simulink model "test_r2_snapshot"  (Simulink 7.9)
settings: Solver=ode45  StartTime=0.0  StopTime=10.0  RelTol=1e-3
libraries: xbsIndex_r4 x545, xps_library x13, casper_library_misc x4, casper_library_scopes x2
(part 1 of 4)
settings Model: Creator=jmanley  LastModifiedBy=jmanley

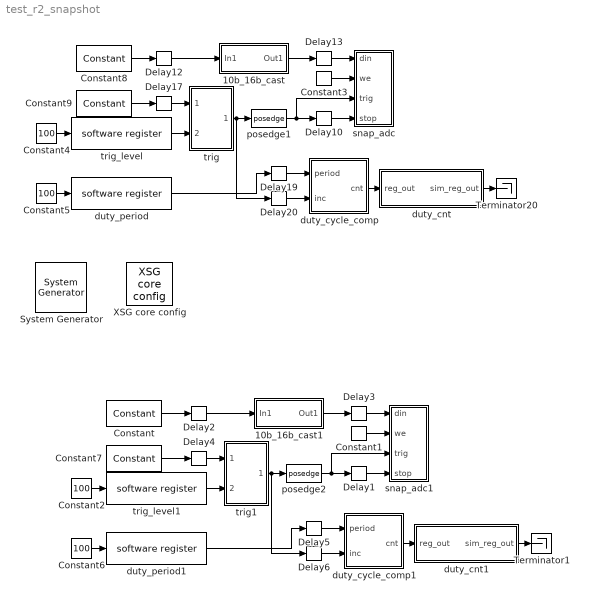
== system test_r2_snapshot ==
  " System Generator" : xbsIndex_r4/ System Generator  Tag=genX  xilinxfamily=virtex5  part=xc5vsx95t  speed=-1  package=ff1136  synthesis_tool=XST  clock_wrapper=Clock Enables  directory=./test_ratt2_snapshot/sysgen  proj_type=Project Navigator  Synth_file=XST Defaults  Impl_file=ISE Defaults  testbench=off  simulink_period=1  sysclk_period=5  dcm_input_clock_period=100  incr_netlist=off  trim_vbits=Everywhere in SubSystem  dbl_ovrd=According to Block Masks  core_generation=According to Block Masks  run_coregen=off  deprecated_control=off  eval_field=0  block_type=sysgen
      settings: block_version=11.4
  10b_16b_cast : Subsystem
  10b_16b_cast1 : Subsystem
  Constant : xbsIndex_r4/Constant  const=0  gui_display_data_type=Fixed-point  arith_type=Unsigned  n_bits=80  bin_pt=0  preci_type=Single  exp_width=8  frac_width=24  explicit_period=on  period=1  equ=P=C  opselect=C  inp2=PCIN>>17  opr=+  inp1=P  carry=CIN  dbl_ovrd=off  block_type=constant
      settings: block_version=11.4
  Constant1 : xbsIndex_r4/Constant  const=1  gui_display_data_type=Fixed-point  arith_type=Boolean  n_bits=1  bin_pt=0  preci_type=Single  exp_width=8  frac_width=24  explicit_period=off  period=1  equ=P=C  opselect=C  inp2=PCIN>>17  opr=+  inp1=P  carry=CIN  dbl_ovrd=off  block_type=constant
      settings: block_version=11.4
  Constant{2,4..6} (4 alike) : Constant  Value=100
  Constant3 : xbsIndex_r4/Constant  const=1  gui_display_data_type=Fixed-point  arith_type=Boolean  n_bits=1  bin_pt=0  preci_type=Single  exp_width=8  frac_width=24  explicit_period=off  period=1  equ=P=C  opselect=C  inp2=PCIN>>17  opr=+  inp1=P  carry=CIN  dbl_ovrd=off  block_type=constant
      settings: block_version=11.4
  Constant7 : xbsIndex_r4/Constant  const=0  gui_display_data_type=Fixed-point  arith_type=Unsigned  n_bits=80  bin_pt=0  preci_type=Single  exp_width=8  frac_width=24  explicit_period=on  period=1  equ=P=C  opselect=C  inp2=PCIN>>17  opr=+  inp1=P  carry=CIN  dbl_ovrd=off  block_type=constant
      settings: block_version=11.4
  Constant8 : xbsIndex_r4/Constant  const=(2^80)-1  gui_display_data_type=Fixed-point  arith_type=Unsigned  n_bits=80  bin_pt=0  preci_type=Single  exp_width=8  frac_width=24  explicit_period=on  period=1  equ=P=C  opselect=C  inp2=PCIN>>17  opr=+  inp1=P  carry=CIN  dbl_ovrd=off  block_type=constant
      settings: block_version=11.4
  Constant9 : xbsIndex_r4/Constant  const=(2^80)-1  gui_display_data_type=Fixed-point  arith_type=Unsigned  n_bits=80  bin_pt=0  preci_type=Single  exp_width=8  frac_width=24  explicit_period=on  period=1  equ=P=C  opselect=C  inp2=PCIN>>17  opr=+  inp1=P  carry=CIN  dbl_ovrd=off  block_type=constant
      settings: block_version=11.4
  Delay{1..6,10,12..13,17,19..20} (12 alike) : xbsIndex_r4/Delay  rst=off  infoeditControl=Selection of Reset will increase slice count due to use of real FFs and instead of SRLs  en=off  latency=2  dbl_ovrd=off  reg_retiming=on  block_type=delay
  Terminator1 : Terminator
  Terminator20 : Terminator
  XSG core config : xps_library/XSG core config  Tag=xps:xsg  hw_sys=ROACH2:sx475t  clk_src=sys_clk  ROACH_clk_src=sys_clk2x  ROACH2_clk_src=sys_clk  clk_rate=225  sample_period=1  synthesis_tool=XST
  duty_cnt : Subsystem  Tag=xps:sw_reg  mask{io_dir=To Processor, arith_type=Unsigned, bitwidth=32, bin_pt=0, sample_period=1, latency=0}
      mask prompts: io_dir "I/O direction"; arith_type "Data Type"; bitwidth "Data bitwidth"; bin_pt "Data binary point"; sample_period "Sample period"
      mask init:
      | gw_name = clear_name(gcb);
      | config.source = str2func('software_register_init');
      | config.toplevel = gcb;
      | xBlock( config, {io_dir, arith_type, bitwidth, bin_pt, ... 
      |     sample_period, gw_name, latency});
      mask StyleString: popup(From Processor|To Processor),popup(Unsigned|Signed  (2's comp)),edit,edit,edit,edit
  duty_cnt1 : Subsystem  Tag=xps:sw_reg  mask{io_dir=To Processor, arith_type=Unsigned, bitwidth=32, bin_pt=0, sample_period=1, latency=0}
      mask prompts: io_dir "I/O direction"; arith_type "Data Type"; bitwidth "Data bitwidth"; bin_pt "Data binary point"; sample_period "Sample period"
      mask init:
      | gw_name = clear_name(gcb);
      | config.source = str2func('software_register_init');
      | config.toplevel = gcb;
      | xBlock( config, {io_dir, arith_type, bitwidth, bin_pt, ... 
      |     sample_period, gw_name, latency});
      mask StyleString: popup(From Processor|To Processor),popup(Unsigned|Signed  (2's comp)),edit,edit,edit,edit
  duty_cycle_comp : Subsystem  mask{chan_bits=12}
      mask prompts: chan_bits "Number of Channels (2^?)"
  duty_cycle_comp1 : Subsystem  mask{chan_bits=12}
      mask prompts: chan_bits "Number of Channels (2^?)"
  duty_period : xps_library/software register  Tag=xps:sw_reg  io_dir=From Processor  arith_type=Unsigned  bitwidth=32  bin_pt=0  sample_period=1  gw_name=test_ratt2_snapshot_duty_period_user_data_out
  duty_period1 : xps_library/software register  Tag=xps:sw_reg  io_dir=From Processor  arith_type=Unsigned  bitwidth=32  bin_pt=0  sample_period=1  gw_name=test_ratt2_snapshot_duty_period1_user_data_out
  posedge1 : casper_library_misc/posedge  Tag=Rising Edge Detector
  posedge2 : casper_library_misc/posedge  Tag=Rising Edge Detector
  snap_adc : Subsystem  AncestorBlock=casper_library_scopes/snapshot  mask(snapshot){storage=bram, dram_dimm=1, dram_clock=200, nsamples=12, data_width=128, offset=on, circap=on, value=off, use_dsp48=on}
      mask prompts: storage "Storage medium"; dram_dimm "DRAM dimm"; dram_clock "DRAM clock rate"; nsamples "Number of Samples (2^?)"; data_width "Data width"; offset "Start delay support"; circap "Circular capture support"; value "Extra value capture support"; use_dsp48 "Use DSP48s to implement counters"
      mask help:
      | Standard snap block, but with the following optional extras;
      |  1) Optionally delay the fabric trigger by a user-specified number of valids.
      |  2) Capture continuously after a trigger until a stop pulse is received. Data is captured into BRAM continuously, with old data being overwritten until a stop command is received. Then stop capturing when memory is filled. This enables you to get some data before and some data after the stop pulse. Use the 'tr_en_cnt' register to determine where you are in your vector. 'Addr' register's MSb now indicates 'busy capturing'.
      |  3) Optionally capture a value on an input port to a register at the same time as the first data sample.
      |  4) Implement counters using DSP48Es to save resources.
      mask init:
      | snapshot_init(gcb, ...
      |     'storage', storage, ...
      |     'dram_dimm', dram_dimm, ...
      |     'dram_clock', dram_clock, ...
      |     'nsamples', nsamples, ...
      |     'data_width', data_width, ...
      |     'offset', offset, ...
      |     'circap', circap, ...
      |     'value', value, ...
      |     'use_dsp48', use_dsp48);
      mask StyleString: popup(bram|dram),popup(1|2|3|4),popup(200|250|266|300|333),edit,popup(8|16|32|64|128),checkbox,checkbox,checkbox,checkbox
      mask CallbackString: snapshot_callback();||||||||
  snap_adc1 : Subsystem  AncestorBlock=casper_library_scopes/snapshot  mask(snapshot){storage=bram, dram_dimm=1, dram_clock=200, nsamples=12, data_width=128, offset=on, circap=on, value=off, use_dsp48=on}
      mask prompts: storage "Storage medium"; dram_dimm "DRAM dimm"; dram_clock "DRAM clock rate"; nsamples "Number of Samples (2^?)"; data_width "Data width"; offset "Start delay support"; circap "Circular capture support"; value "Extra value capture support"; use_dsp48 "Use DSP48s to implement counters"
      mask help:
      | Standard snap block, but with the following optional extras;
      |  1) Optionally delay the fabric trigger by a user-specified number of valids.
      |  2) Capture continuously after a trigger until a stop pulse is received. Data is captured into BRAM continuously, with old data being overwritten until a stop command is received. Then stop capturing when memory is filled. This enables you to get some data before and some data after the stop pulse. Use the 'tr_en_cnt' register to determine where you are in your vector. 'Addr' register's MSb now indicates 'busy capturing'.
      |  3) Optionally capture a value on an input port to a register at the same time as the first data sample.
      |  4) Implement counters using DSP48Es to save resources.
      mask init: same as test_r2_snapshot/snap_adc
      mask StyleString: popup(bram|dram),popup(1|2|3|4),popup(200|250|266|300|333),edit,popup(8|16|32|64|128),checkbox,checkbox,checkbox,checkbox
      mask CallbackString: snapshot_callback();||||||||
  trig : Subsystem
  trig1 : Subsystem
  trig_level : xps_library/software register  Tag=xps:sw_reg  io_dir=From Processor  arith_type=Unsigned  bitwidth=32  bin_pt=0  sample_period=1  gw_name=test_ratt2_snapshot_trig_level_user_data_out
  trig_level1 : xps_library/software register  Tag=xps:sw_reg  io_dir=From Processor  arith_type=Unsigned  bitwidth=32  bin_pt=0  sample_period=1  gw_name=test_ratt2_snapshot_trig_level1_user_data_out
  wires:
  Constant4/1 -> trig_level/1
  Constant9/1 -> Delay17/1
  trig/1(trig) -> posedge1/1, Delay20/1
  trig_level/1 -> trig/2(trig_pnt)
  Delay17/1 -> trig/1(adc_data)
  posedge1/1 -> Delay10/1, snap_adc/3(trig)
  Delay10/1 -> snap_adc/4(stop)
  Constant5/1 -> duty_period/1
  duty_period/1 -> Delay19/1
  duty_cnt/1(sim_reg_out) -> Terminator20/1
  duty_cycle_comp/1(cnt) -> duty_cnt/1(reg_out)
  Delay19/1 -> duty_cycle_comp/1(period)
  Delay20/1 -> duty_cycle_comp/2(inc)
  Constant3/1 -> snap_adc/2(we)
  Constant8/1 -> Delay12/1
  Delay12/1 -> 10b_16b_cast/1(In1)
  10b_16b_cast/1(Out1) -> Delay13/1
  Delay13/1 -> snap_adc/1(din)
  Constant2/1 -> trig_level1/1
  Constant7/1 -> Delay4/1
  trig1/1(trig) -> Delay6/1, posedge2/1
  trig_level1/1 -> trig1/2(trig_pnt)
  Delay4/1 -> trig1/1(adc_data)
  posedge2/1 -> snap_adc1/3(trig), Delay1/1
  Delay1/1 -> snap_adc1/4(stop)
  Constant6/1 -> duty_period1/1
  duty_period1/1 -> Delay5/1
  duty_cnt1/1(sim_reg_out) -> Terminator1/1
  duty_cycle_comp1/1(cnt) -> duty_cnt1/1(reg_out)
  Delay5/1 -> duty_cycle_comp1/1(period)
  Delay6/1 -> duty_cycle_comp1/2(inc)
  Constant1/1 -> snap_adc1/2(we)
  Constant/1 -> Delay2/1
  Delay2/1 -> 10b_16b_cast1/1(In1)
  10b_16b_cast1/1(Out1) -> Delay3/1
  Delay3/1 -> snap_adc1/1(din)

== system test_r2_snapshot/10b_16b_cast ==
  In1 : Inport
  Convert{,1..7} (8 alike) : xbsIndex_r4/Convert  gui_display_data_type=Fixed-point  arith_type="Signed  (2's comp)"  n_bits=16  bin_pt=0  float_type=Single  exp_bits=8  fraction_bits=24  quantization=Truncate  overflow=Wrap  en=off  latency=0  dbl_ovrd=off  pipeline=off  block_type=convert
  adc0_bus_create1 : Subsystem  AncestorBlock=casper_library_flow_control/bus_create  mask(bus_create){inputNum=8}
      mask prompts: inputNum "Number of inputs:"
      mask init:
      | bus_create_init(gcb,...
      |     'inputNum', inputNum);
  bus_expand2 : Subsystem  AncestorBlock=casper_library_flow_control/bus_expand  mask(bus_expand){mode=divisions of equal size, outputNum=8, outputWidth=10, outputBinaryPt=0, outputArithmeticType=1, outputToWorkspace=off, variablePrefix=out, outputToModelAsWell=on}
      mask prompts: outputNum "Number of outputs:"; outputWidth "Output width:"; outputBinaryPt "Output binary point position:"; outputArithmeticType "Output arithmetic type: (Unsigned=0, Signed=1, Boolean=2)"; outputToWorkspace "Output to workspace?"; variablePrefix "Variable name prefix:"; outputToModelAsWell "Output to model as well?"
      mask help:
      | Expands a 'bus' made using a bus_create or Xilinx
      | concat block.
      | The input will be divided into the specified number
      | of outputs with the specified arithmetic types.
      | Divisions are made from most significant bit.
      mask init:
      | bus_expand_init(gcb,...
      |     'mode', mode, ...
      |     'outputNum', outputNum, ...
      |     'outputWidth', outputWidth, ...
      |     'outputBinaryPt', outputBinaryPt, ...
      |     'outputArithmeticType', outputArithmeticType, ...
      |     'outputToWorkspace', outputToWorkspace, ...
      |     'variablePrefix', variablePrefix, ...
      |     'outputToModelAsWell', outputToModelAsWell);
      settings: AttributesFormatString=8 outputs
      mask StyleString: popup(divisions of equal size|divisions of arbitrary size),edit,edit,edit,edit,checkbox,edit,checkbox
      mask CallbackString: bus_expand_callback();||bus_expand_callback();|||bus_expand_callback();||
  Out1 : Outport
  wires:
  bus_expand2/1(msb_out8) -> Convert/1
  bus_expand2/2(out7) -> Convert1/1
  bus_expand2/3(out6) -> Convert2/1
  bus_expand2/4(out5) -> Convert3/1
  bus_expand2/5(out4) -> Convert4/1
  bus_expand2/6(out3) -> Convert5/1
  bus_expand2/7(out2) -> Convert6/1
  bus_expand2/8(lsb_out1) -> Convert7/1
  Convert/1 -> adc0_bus_create1/1(in1)
  Convert1/1 -> adc0_bus_create1/2(in2)
  Convert2/1 -> adc0_bus_create1/3(in3)
  Convert3/1 -> adc0_bus_create1/4(in4)
  Convert4/1 -> adc0_bus_create1/5(in5)
  Convert5/1 -> adc0_bus_create1/6(in6)
  Convert6/1 -> adc0_bus_create1/7(in7)
  Convert7/1 -> adc0_bus_create1/8(in8)
  adc0_bus_create1/1(bus_out) -> Out1/1
  In1/1 -> bus_expand2/1(bus_in)

== system test_r2_snapshot/10b_16b_cast1 ==
  In1 : Inport
  Convert{,1..7} (8 alike) : xbsIndex_r4/Convert  gui_display_data_type=Fixed-point  arith_type="Signed  (2's comp)"  n_bits=16  bin_pt=0  float_type=Single  exp_bits=8  fraction_bits=24  quantization=Truncate  overflow=Wrap  en=off  latency=0  dbl_ovrd=off  pipeline=off  block_type=convert
  adc0_bus_create1 : Subsystem  AncestorBlock=casper_library_flow_control/bus_create  mask(bus_create){inputNum=8}
      mask prompts: inputNum "Number of inputs:"
      mask init:
      | bus_create_init(gcb,...
      |     'inputNum', inputNum);
  bus_expand2 : Subsystem  AncestorBlock=casper_library_flow_control/bus_expand  mask(bus_expand){mode=divisions of equal size, outputNum=8, outputWidth=10, outputBinaryPt=0, outputArithmeticType=1, outputToWorkspace=off, variablePrefix=out, outputToModelAsWell=on}
      mask prompts: outputNum "Number of outputs:"; outputWidth "Output width:"; outputBinaryPt "Output binary point position:"; outputArithmeticType "Output arithmetic type: (Unsigned=0, Signed=1, Boolean=2)"; outputToWorkspace "Output to workspace?"; variablePrefix "Variable name prefix:"; outputToModelAsWell "Output to model as well?"
      mask help:
      | Expands a 'bus' made using a bus_create or Xilinx
      | concat block.
      | The input will be divided into the specified number
      | of outputs with the specified arithmetic types.
      | Divisions are made from most significant bit.
      mask init: same as test_r2_snapshot/10b_16b_cast/bus_expand2
      settings: AttributesFormatString=8 outputs
      mask StyleString: popup(divisions of equal size|divisions of arbitrary size),edit,edit,edit,edit,checkbox,edit,checkbox
      mask CallbackString: bus_expand_callback();||bus_expand_callback();|||bus_expand_callback();||
  Out1 : Outport
  wires:
  In1/1 -> bus_expand2/1(bus_in)
  adc0_bus_create1/1(bus_out) -> Out1/1
  Convert7/1 -> adc0_bus_create1/8(in8)
  Convert6/1 -> adc0_bus_create1/7(in7)
  Convert5/1 -> adc0_bus_create1/6(in6)
  Convert4/1 -> adc0_bus_create1/5(in5)
  Convert3/1 -> adc0_bus_create1/4(in4)
  Convert2/1 -> adc0_bus_create1/3(in3)
  Convert1/1 -> adc0_bus_create1/2(in2)
  Convert/1 -> adc0_bus_create1/1(in1)
  bus_expand2/8(lsb_out1) -> Convert7/1
  bus_expand2/7(out2) -> Convert6/1
  bus_expand2/6(out3) -> Convert5/1
  bus_expand2/5(out4) -> Convert4/1
  bus_expand2/4(out5) -> Convert3/1
  bus_expand2/3(out6) -> Convert2/1
  bus_expand2/2(out7) -> Convert1/1
  bus_expand2/1(msb_out8) -> Convert/1

== system test_r2_snapshot/duty_cnt ==
  reg_out : Inport
  convert : xbsIndex_r4/Convert  gui_display_data_type=Fixed-point  arith_type=Unsigned  n_bits=32  bin_pt=0  float_type=Single  exp_bits=8  fraction_bits=24  quantization=Truncate  overflow=Wrap  en=off  latency=0  dbl_ovrd=off  pipeline=off  block_type=convert
  test_ratt2_snapshot_duty_cnt_user_data_in : xbsIndex_r4/Gateway Out  inherit_from_input=off  hdl_port=on  timing_constraint=None  locs_specified=off  LOCs={}  UseAsDAC=off  DACChannel='1'  block_type=gatewayout
  sim_reg_out : Outport
  wires:
  reg_out/1 -> convert/1
  convert/1 -> test_ratt2_snapshot_duty_cnt_user_data_in/1
  test_ratt2_snapshot_duty_cnt_user_data_in/1 -> sim_reg_out/1

== system test_r2_snapshot/duty_cnt1 ==
  reg_out : Inport
  convert : xbsIndex_r4/Convert  gui_display_data_type=Fixed-point  arith_type=Unsigned  n_bits=32  bin_pt=0  float_type=Single  exp_bits=8  fraction_bits=24  quantization=Truncate  overflow=Wrap  en=off  latency=0  dbl_ovrd=off  pipeline=off  block_type=convert
  test_ratt2_snapshot_duty_cnt1_user_data_in : xbsIndex_r4/Gateway Out  inherit_from_input=off  hdl_port=on  timing_constraint=None  locs_specified=off  LOCs={}  UseAsDAC=off  DACChannel='1'  block_type=gatewayout
  sim_reg_out : Outport
  wires:
  reg_out/1 -> convert/1
  convert/1 -> test_ratt2_snapshot_duty_cnt1_user_data_in/1
  test_ratt2_snapshot_duty_cnt1_user_data_in/1 -> sim_reg_out/1

== system test_r2_snapshot/duty_cycle_comp ==
  period : Inport
  inc : Inport  Port=2
  AddSub : xbsIndex_r4/AddSub  mode=Subtraction  use_carryin=off  use_carryout=off  en=off  latency=1  precision=User Defined  arith_type=Unsigned  n_bits=32  bin_pt=0  quantization=Truncate  overflow=Wrap  dbl_ovrd=off  use_behavioral_HDL=off  hw_selection=DSP48  pipelined=on  block_type=addsub
  Constant2 : xbsIndex_r4/Constant  const=2  gui_display_data_type=Fixed-point  arith_type=Unsigned  n_bits=2  bin_pt=0  preci_type=Single  exp_width=8  frac_width=24  explicit_period=on  period=1  equ=P=C  opselect=C  inp2=PCIN>>17  opr=+  inp1=P  carry=CIN  dbl_ovrd=off  block_type=constant
  Delay1 : xbsIndex_r4/Delay  rst=off  infoeditControl=Selection of Reset will increase slice count due to use of real FFs and instead of SRLs  en=off  latency=1  dbl_ovrd=off  reg_retiming=on  block_type=delay
      settings: xl_area=[0, 0, 0, 0, 0, 0, 0]
  Delay2 : xbsIndex_r4/Delay  rst=off  infoeditControl=Selection of Reset will increase slice count due to use of real FFs and instead of SRLs  en=off  latency=1  dbl_ovrd=off  reg_retiming=on  block_type=delay
      settings: xl_area=[0, 0, 0, 0, 0, 0, 0]
  Register : xbsIndex_r4/Register  init=0  rst=off  en=on  dbl_ovrd=off  block_type=register
      settings: xl_area=[0, 0, 0, 0, 0, 0, 0]
  Relational5 : xbsIndex_r4/Relational  mode=a>=b  en=off  latency=1  dbl_ovrd=off  block_type=relational
      settings: xl_area=[0, 0, 0, 0, 0, 0, 0]  block_version=10.1.3
  Shift : xbsIndex_r4/Shift  shift_dir=Left  shift_bits=chan_bits  en=off  latency=0  precision=Full  arith_type="Signed  (2's comp)"  n_bits=8  bin_pt=2  quantization=Truncate  overflow=Wrap  dbl_ovrd=off  block_type=shift
      settings: xl_area=[0, 0, 0, 0, 0, 0, 0]  block_version=10.1.3
  cntr : xbsIndex_r4/Counter  cnt_type=Free Running  cnt_to=Inf  operation=Up  start_count=1  cnt_by_val=1  arith_type=Unsigned  n_bits=32  bin_pt=0  load_pin=off  rst=on  en=off  explicit_period=on  period=1  dbl_ovrd=off  use_behavioral_HDL=on  implementation=Fabric  use_rpm=on  block_type=counter
      settings: xl_area=[0, 0, 0, 0, 0, 0, 0]
  cntr1 : xbsIndex_r4/Counter  cnt_type=Free Running  cnt_to=Inf  operation=Up  start_count=1  cnt_by_val=1  arith_type=Unsigned  n_bits=32  bin_pt=0  load_pin=off  rst=on  en=on  explicit_period=on  period=1  dbl_ovrd=off  use_behavioral_HDL=on  implementation=Fabric  use_rpm=on  block_type=counter
      settings: xl_area=[0, 0, 0, 0, 0, 0, 0]
  posedge2 : Subsystem  Tag=Rising Edge Detector
  cnt : Outport
  wires:
  Constant2/1 -> AddSub/2
  AddSub/1 -> Delay2/1
  Shift/1 -> AddSub/1
  Delay1/1 -> posedge2/1(In)
  Relational5/1 -> Delay1/1, cntr/1
  period/1 -> Shift/1
  posedge2/1(Out) -> cntr1/1, Register/2
  Delay2/1 -> Relational5/2
  cntr/1 -> Relational5/1
  inc/1 -> cntr1/2
  cntr1/1 -> Register/1
  Register/1 -> cnt/1

== system test_r2_snapshot/duty_cycle_comp1 ==
  period : Inport
  inc : Inport  Port=2
  AddSub : xbsIndex_r4/AddSub  mode=Subtraction  use_carryin=off  use_carryout=off  en=off  latency=1  precision=User Defined  arith_type=Unsigned  n_bits=32  bin_pt=0  quantization=Truncate  overflow=Wrap  dbl_ovrd=off  use_behavioral_HDL=off  hw_selection=DSP48  pipelined=on  block_type=addsub
  Constant2 : xbsIndex_r4/Constant  const=2  gui_display_data_type=Fixed-point  arith_type=Unsigned  n_bits=2  bin_pt=0  preci_type=Single  exp_width=8  frac_width=24  explicit_period=on  period=1  equ=P=C  opselect=C  inp2=PCIN>>17  opr=+  inp1=P  carry=CIN  dbl_ovrd=off  block_type=constant
  Delay1 : xbsIndex_r4/Delay  rst=off  infoeditControl=Selection of Reset will increase slice count due to use of real FFs and instead of SRLs  en=off  latency=1  dbl_ovrd=off  reg_retiming=on  block_type=delay
      settings: xl_area=[0, 0, 0, 0, 0, 0, 0]
  Delay2 : xbsIndex_r4/Delay  rst=off  infoeditControl=Selection of Reset will increase slice count due to use of real FFs and instead of SRLs  en=off  latency=1  dbl_ovrd=off  reg_retiming=on  block_type=delay
      settings: xl_area=[0, 0, 0, 0, 0, 0, 0]
  Register : xbsIndex_r4/Register  init=0  rst=off  en=on  dbl_ovrd=off  block_type=register
      settings: xl_area=[0, 0, 0, 0, 0, 0, 0]
  Relational5 : xbsIndex_r4/Relational  mode=a>=b  en=off  latency=1  dbl_ovrd=off  block_type=relational
      settings: xl_area=[0, 0, 0, 0, 0, 0, 0]  block_version=10.1.3
  Shift : xbsIndex_r4/Shift  shift_dir=Left  shift_bits=chan_bits  en=off  latency=0  precision=Full  arith_type="Signed  (2's comp)"  n_bits=8  bin_pt=2  quantization=Truncate  overflow=Wrap  dbl_ovrd=off  block_type=shift
      settings: xl_area=[0, 0, 0, 0, 0, 0, 0]  block_version=10.1.3
  cntr : xbsIndex_r4/Counter  cnt_type=Free Running  cnt_to=Inf  operation=Up  start_count=1  cnt_by_val=1  arith_type=Unsigned  n_bits=32  bin_pt=0  load_pin=off  rst=on  en=off  explicit_period=on  period=1  dbl_ovrd=off  use_behavioral_HDL=on  implementation=Fabric  use_rpm=on  block_type=counter
      settings: xl_area=[0, 0, 0, 0, 0, 0, 0]
  cntr1 : xbsIndex_r4/Counter  cnt_type=Free Running  cnt_to=Inf  operation=Up  start_count=1  cnt_by_val=1  arith_type=Unsigned  n_bits=32  bin_pt=0  load_pin=off  rst=on  en=on  explicit_period=on  period=1  dbl_ovrd=off  use_behavioral_HDL=on  implementation=Fabric  use_rpm=on  block_type=counter
      settings: xl_area=[0, 0, 0, 0, 0, 0, 0]
  posedge2 : Subsystem  Tag=Rising Edge Detector
  cnt : Outport
  wires:
  Register/1 -> cnt/1
  cntr1/1 -> Register/1
  inc/1 -> cntr1/2
  cntr/1 -> Relational5/1
  Delay2/1 -> Relational5/2
  posedge2/1(Out) -> Register/2, cntr1/1
  period/1 -> Shift/1
  Relational5/1 -> cntr/1, Delay1/1
  Delay1/1 -> posedge2/1(In)
  Shift/1 -> AddSub/1
  AddSub/1 -> Delay2/1
  Constant2/1 -> AddSub/2

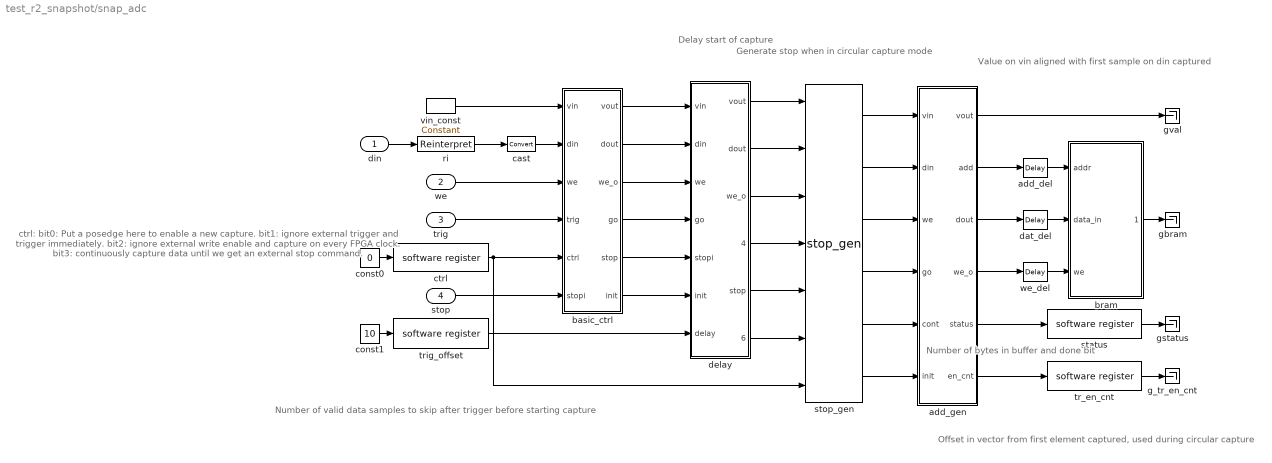
== system test_r2_snapshot/snap_adc ==
  note: Generate stop
      | when in circular
      | capture mode
  note: Delay start
      | of capture
  note: ctrl:
      | bit0: Put a posedge here
      |         to enable a new capture.
      | bit1: ignore external trigger
      |         and trigger immediately.
      | bit2: ignore external write
      |         enable and capture on
      |         every FPGA clock.
      | bit3: continuously capture
      |         data until we get an
      |         external stop command.
  note: Offset in vector
      | from first element
      | captured, used
      | during circular capture
  note: Number of
      | bytes in
      | buffer and
      | done bit
  note: Number of valid
      | data samples to
      | skip after trigger
      | before starting
      | capture
  note: Value on vin
      | aligned with
      | first sample on
      | din captured
  din : Inport
  we : Inport  Port=2
  trig : Inport  Port=3
  stop : Inport  Port=4
  add_del : xbsIndex_r4/Delay  rst=off  infoeditControl=Selection of Reset will increase slice count due to use of real FFs and instead of SRLs  en=off  latency=1  dbl_ovrd=off  reg_retiming=off  block_type=delay
  add_gen : Subsystem  AncestorBlock=casper_library_scopes/snapshot/add_gen  mask{counter_size=32, increment=16, nsamples=12, burst_size=0, use_dsp48=on}
      mask prompts: counter_size "Address counter size (2^?)"; increment "Address counter increment"; nsamples "Number of samples (2^?)"; burst_size "Burst size (2^?)"; use_dsp48 "dsp48 counter/s"
      mask init:
      | set_param(gcb,'LinkStatus','inactive');
      | if strcmp(use_dsp48,'on'),
      |     set_param([gcb,'/add_gen'],'implementation','DSP48');
      | else
      |     set_param([gcb,'/add_gen'],'implementation','Fabric');
      | end
  basic_ctrl : Subsystem  AncestorBlock=casper_library_scopes/snapshot/basic_ctrl  mask{dram=off, data_width=128}
      mask prompts: data_width "data width"
      mask init:
      | set_param(gcb,'LinkStatus','inactive');
      | set_param([gcb,'/dram_munge'], 'dram', dram);
  bram : Subsystem  Tag=xps:bram  AncestorBlock=xps_library/Shared BRAM  mask{arith_type=Unsigned, addr_width=12, data_width=128, data_bin_pt=0, init_vals=[0:2^10-1], sample_rate=1}
      mask prompts: arith_type "Output Data Type"; addr_width "Address width"; data_width "Data Width"; data_bin_pt "Data Binary Point"; init_vals "Initial 32-bit values (simulation only)"; sample_rate "Sample rate"
      mask init:
      | shared_bram_mask;
      mask StyleString: popup(Unsigned|Signed  (2's comp)),edit,popup(8|16|32|64|128),edit,edit,edit
  cast : xbsIndex_r4/Convert  gui_display_data_type=Fixed-point  arith_type=Unsigned  n_bits=128  bin_pt=0  float_type=Single  exp_bits=8  fraction_bits=24  quantization=Truncate  overflow=Wrap  en=off  latency=0  dbl_ovrd=off  pipeline=off  block_type=convert
  const0 : Constant  Value=0
  const1 : Constant  Value=10
  ctrl : xps_library/software register  Tag=xps:sw_reg  io_dir=From Processor  arith_type=Unsigned  bitwidth=32  bin_pt=0  sample_period=1  gw_name=test_ratt2_snapshot_snap_adc_ctrl_user_data_out
  dat_del : xbsIndex_r4/Delay  rst=off  infoeditControl=Selection of Reset will increase slice count due to use of real FFs and instead of SRLs  en=off  latency=1  dbl_ovrd=off  reg_retiming=off  block_type=delay
  delay : Subsystem  AncestorBlock=casper_library_scopes/snapshot/delay  mask{use_dsp48=on, word_size=16}
      mask prompts: use_dsp48 "dsp48 counter/s"; word_size "word byte size?"
      mask init:
      | set_param(gcb,'LinkStatus','inactive');
      | if strcmp(use_dsp48,'on'),
      |     set_param([gcb,'/counter'],'implementation','DSP48');
      | else
      |     set_param([gcb,'/counter'],'implementation','Fabric');
      | end
  g_tr_en_cnt : Terminator
  gbram : Terminator
  gstatus : Terminator
  gval : Terminator
  ri : xbsIndex_r4/Reinterpret  force_arith_type=on  arith_type=Unsigned  force_bin_pt=on  bin_pt=0  block_type=reinterpret
  status : xps_library/software register  Tag=xps:sw_reg  io_dir=To Processor  arith_type=Unsigned  bitwidth=32  bin_pt=0  sample_period=1  gw_name=test_ratt2_snapshot_snap_adc_status_user_data_in
  stop_gen : casper_library_scopes/snapshot/stop_gen
  tr_en_cnt : xps_library/software register  Tag=xps:sw_reg  io_dir=To Processor  arith_type=Unsigned  bitwidth=32  bin_pt=0  sample_period=1  gw_name=test_ratt2_snapshot_snap_adc_tr_en_cnt_user_data_in
  trig_offset : xps_library/software register  Tag=xps:sw_reg  io_dir=From Processor  arith_type=Unsigned  bitwidth=32  bin_pt=0  sample_period=1  gw_name=test_ratt2_snapshot_snap_adc_trig_offset_user_data_out
  vin_const : xbsIndex_r4/Constant  const=0  gui_display_data_type=Fixed-point  arith_type=Boolean  n_bits=16  bin_pt=14  preci_type=Single  exp_width=8  frac_width=24  explicit_period=on  period=1  equ=P=C  opselect=C  inp2=PCIN>>17  opr=+  inp1=P  carry=CIN  dbl_ovrd=off  block_type=constant
  we_del : xbsIndex_r4/Delay  rst=off  infoeditControl=Selection of Reset will increase slice count due to use of real FFs and instead of SRLs  en=off  latency=1  dbl_ovrd=off  reg_retiming=off  block_type=delay
  wires:
  din/1 -> ri/1
  ri/1 -> cast/1
  cast/1 -> basic_ctrl/2(din)
  we/1 -> basic_ctrl/3(we)
  trig/1 -> basic_ctrl/4(trig)
  stop/1 -> basic_ctrl/6(stopi)
  const0/1 -> ctrl/1
  ctrl/1 -> basic_ctrl/5(ctrl), stop_gen/7
  const1/1 -> trig_offset/1
  basic_ctrl/1(vout) -> delay/1(vin)
  basic_ctrl/2(dout) -> delay/2(din)
  basic_ctrl/3(we_o) -> delay/3(we)
  basic_ctrl/4(go) -> delay/4(go)
  basic_ctrl/5(stop) -> delay/5(stopi)
  basic_ctrl/6(init) -> delay/6(init)
  trig_offset/1 -> delay/7(delay)
  delay/1(vout) -> stop_gen/1
  delay/2(dout) -> stop_gen/2
  delay/3(we_o) -> stop_gen/3
  delay/4(del_go) -> stop_gen/4
  delay/5(stop) -> stop_gen/5
  delay/6(del_init) -> stop_gen/6
  tr_en_cnt/1 -> g_tr_en_cnt/1
  stop_gen/1 -> add_gen/1(vin)
  stop_gen/2 -> add_gen/2(din)
  stop_gen/3 -> add_gen/3(we)
  stop_gen/4 -> add_gen/4(go)
  stop_gen/5 -> add_gen/5(cont)
  stop_gen/6 -> add_gen/6(init)
  add_gen/5(status) -> status/1
  status/1 -> gstatus/1
  vin_const/1 -> basic_ctrl/1(vin)
  add_gen/1(vout) -> gval/1
  add_gen/6(en_cnt) -> tr_en_cnt/1
  add_gen/2(add) -> add_del/1
  add_gen/3(dout) -> dat_del/1
  add_gen/4(we_o) -> we_del/1
  add_del/1 -> bram/1(addr)
  dat_del/1 -> bram/2(data_in)
  we_del/1 -> bram/3(we)
  bram/1(data_out) -> gbram/1

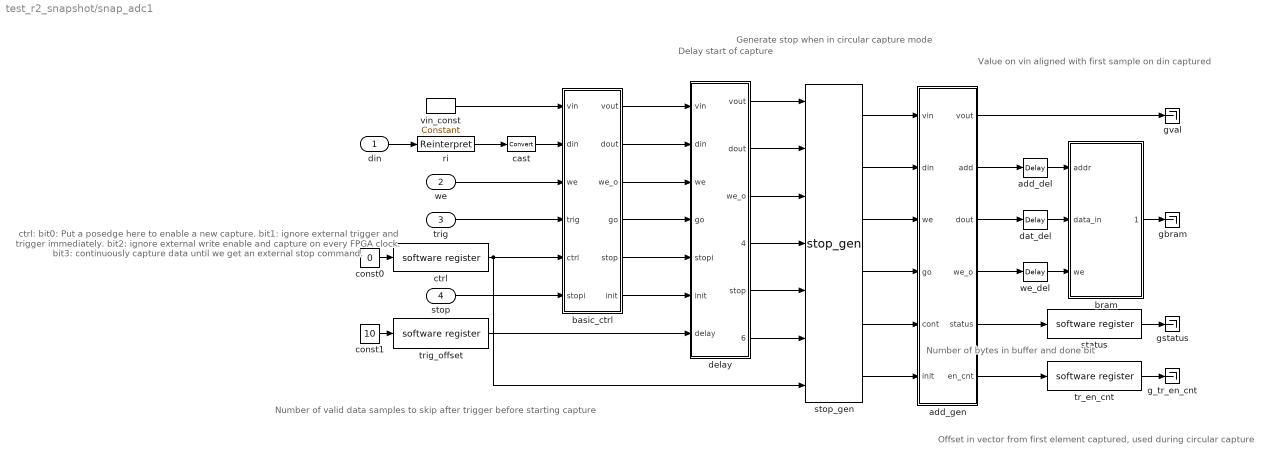
== system test_r2_snapshot/snap_adc1 ==
  note: Value on vin
      | aligned with
      | first sample on
      | din captured
  note: Number of valid
      | data samples to
      | skip after trigger
      | before starting
      | capture
  note: Number of
      | bytes in
      | buffer and
      | done bit
  note: Offset in vector
      | from first element
      | captured, used
      | during circular capture
  note: ctrl:
      | bit0: Put a posedge here
      |         to enable a new capture.
      | bit1: ignore external trigger
      |         and trigger immediately.
      | bit2: ignore external write
      |         enable and capture on
      |         every FPGA clock.
      | bit3: continuously capture
      |         data until we get an
      |         external stop command.
  note: Delay start
      | of capture
  note: Generate stop
      | when in circular
      | capture mode
  din : Inport
  we : Inport  Port=2
  trig : Inport  Port=3
  stop : Inport  Port=4
  add_del : xbsIndex_r4/Delay  rst=off  infoeditControl=Selection of Reset will increase slice count due to use of real FFs and instead of SRLs  en=off  latency=1  dbl_ovrd=off  reg_retiming=off  block_type=delay
  add_gen : Subsystem  AncestorBlock=casper_library_scopes/snapshot/add_gen  mask{counter_size=32, increment=16, nsamples=12, burst_size=0, use_dsp48=on}
      mask prompts: counter_size "Address counter size (2^?)"; increment "Address counter increment"; nsamples "Number of samples (2^?)"; burst_size "Burst size (2^?)"; use_dsp48 "dsp48 counter/s"
      mask init:
      | set_param(gcb,'LinkStatus','inactive');
      | if strcmp(use_dsp48,'on'),
      |     set_param([gcb,'/add_gen'],'implementation','DSP48');
      | else
      |     set_param([gcb,'/add_gen'],'implementation','Fabric');
      | end
  basic_ctrl : Subsystem  AncestorBlock=casper_library_scopes/snapshot/basic_ctrl  mask{dram=off, data_width=128}
      mask prompts: data_width "data width"
      mask init:
      | set_param(gcb,'LinkStatus','inactive');
      | set_param([gcb,'/dram_munge'], 'dram', dram);
  bram : Subsystem  Tag=xps:bram  AncestorBlock=xps_library/Shared BRAM  mask{arith_type=Unsigned, addr_width=12, data_width=128, data_bin_pt=0, init_vals=[0:2^10-1], sample_rate=1}
      mask prompts: arith_type "Output Data Type"; addr_width "Address width"; data_width "Data Width"; data_bin_pt "Data Binary Point"; init_vals "Initial 32-bit values (simulation only)"; sample_rate "Sample rate"
      mask init:
      | shared_bram_mask;
      mask StyleString: popup(Unsigned|Signed  (2's comp)),edit,popup(8|16|32|64|128),edit,edit,edit
  cast : xbsIndex_r4/Convert  gui_display_data_type=Fixed-point  arith_type=Unsigned  n_bits=128  bin_pt=0  float_type=Single  exp_bits=8  fraction_bits=24  quantization=Truncate  overflow=Wrap  en=off  latency=0  dbl_ovrd=off  pipeline=off  block_type=convert
  const0 : Constant  Value=0
  const1 : Constant  Value=10
  ctrl : xps_library/software register  Tag=xps:sw_reg  io_dir=From Processor  arith_type=Unsigned  bitwidth=32  bin_pt=0  sample_period=1  gw_name=test_ratt2_snapshot_snap_adc1_ctrl_user_data_out
  dat_del : xbsIndex_r4/Delay  rst=off  infoeditControl=Selection of Reset will increase slice count due to use of real FFs and instead of SRLs  en=off  latency=1  dbl_ovrd=off  reg_retiming=off  block_type=delay
  delay : Subsystem  AncestorBlock=casper_library_scopes/snapshot/delay  mask{use_dsp48=on, word_size=16}
      mask prompts: use_dsp48 "dsp48 counter/s"; word_size "word byte size?"
      mask init:
      | set_param(gcb,'LinkStatus','inactive');
      | if strcmp(use_dsp48,'on'),
      |     set_param([gcb,'/counter'],'implementation','DSP48');
      | else
      |     set_param([gcb,'/counter'],'implementation','Fabric');
      | end
  g_tr_en_cnt : Terminator
  gbram : Terminator
  gstatus : Terminator
  gval : Terminator
  ri : xbsIndex_r4/Reinterpret  force_arith_type=on  arith_type=Unsigned  force_bin_pt=on  bin_pt=0  block_type=reinterpret
  status : xps_library/software register  Tag=xps:sw_reg  io_dir=To Processor  arith_type=Unsigned  bitwidth=32  bin_pt=0  sample_period=1  gw_name=test_ratt2_snapshot_snap_adc1_status_user_data_in
  stop_gen : casper_library_scopes/snapshot/stop_gen
  tr_en_cnt : xps_library/software register  Tag=xps:sw_reg  io_dir=To Processor  arith_type=Unsigned  bitwidth=32  bin_pt=0  sample_period=1  gw_name=test_ratt2_snapshot_snap_adc1_tr_en_cnt_user_data_in
  trig_offset : xps_library/software register  Tag=xps:sw_reg  io_dir=From Processor  arith_type=Unsigned  bitwidth=32  bin_pt=0  sample_period=1  gw_name=test_ratt2_snapshot_snap_adc1_trig_offset_user_data_out
  vin_const : xbsIndex_r4/Constant  const=0  gui_display_data_type=Fixed-point  arith_type=Boolean  n_bits=16  bin_pt=14  preci_type=Single  exp_width=8  frac_width=24  explicit_period=on  period=1  equ=P=C  opselect=C  inp2=PCIN>>17  opr=+  inp1=P  carry=CIN  dbl_ovrd=off  block_type=constant
  we_del : xbsIndex_r4/Delay  rst=off  infoeditControl=Selection of Reset will increase slice count due to use of real FFs and instead of SRLs  en=off  latency=1  dbl_ovrd=off  reg_retiming=off  block_type=delay
  wires:
  bram/1(data_out) -> gbram/1
  we_del/1 -> bram/3(we)
  dat_del/1 -> bram/2(data_in)
  add_del/1 -> bram/1(addr)
  add_gen/4(we_o) -> we_del/1
  add_gen/3(dout) -> dat_del/1
  add_gen/2(add) -> add_del/1
  add_gen/6(en_cnt) -> tr_en_cnt/1
  add_gen/1(vout) -> gval/1
  vin_const/1 -> basic_ctrl/1(vin)
  status/1 -> gstatus/1
  add_gen/5(status) -> status/1
  stop_gen/6 -> add_gen/6(init)
  stop_gen/5 -> add_gen/5(cont)
  stop_gen/4 -> add_gen/4(go)
  stop_gen/3 -> add_gen/3(we)
  stop_gen/2 -> add_gen/2(din)
  stop_gen/1 -> add_gen/1(vin)
  tr_en_cnt/1 -> g_tr_en_cnt/1
  delay/6(del_init) -> stop_gen/6
  delay/5(stop) -> stop_gen/5
  delay/4(del_go) -> stop_gen/4
  delay/3(we_o) -> stop_gen/3
  delay/2(dout) -> stop_gen/2
  delay/1(vout) -> stop_gen/1
  trig_offset/1 -> delay/7(delay)
  basic_ctrl/6(init) -> delay/6(init)
  basic_ctrl/5(stop) -> delay/5(stopi)
  basic_ctrl/4(go) -> delay/4(go)
  basic_ctrl/3(we_o) -> delay/3(we)
  basic_ctrl/2(dout) -> delay/2(din)
  basic_ctrl/1(vout) -> delay/1(vin)
  const1/1 -> trig_offset/1
  ctrl/1 -> stop_gen/7, basic_ctrl/5(ctrl)
  const0/1 -> ctrl/1
  stop/1 -> basic_ctrl/6(stopi)
  trig/1 -> basic_ctrl/4(trig)
  we/1 -> basic_ctrl/3(we)
  cast/1 -> basic_ctrl/2(din)
  ri/1 -> cast/1
  din/1 -> ri/1

== system test_r2_snapshot/trig ==
  adc_data : Inport
  trig_pnt : Inport  Port=2
  Delay17 : xbsIndex_r4/Delay  rst=off  infoeditControl=Selection of Reset will increase slice count due to use of real FFs and instead of SRLs  en=off  latency=2  dbl_ovrd=off  reg_retiming=on  block_type=delay
  Logical1 : xbsIndex_r4/Logical  logical_function=OR  inputs=8  en=off  latency=2  precision=Full  arith_type=Unsigned  n_bits=16  bin_pt=0  align_bp=on  dbl_ovrd=off  block_type=logical
  Mult : xbsIndex_r4/Mult  precision=Full  arith_type=Unsigned  n_bits=16  bin_pt=14  quantization=Truncate  overflow=Saturate  en=off  latency=4  dbl_ovrd=off  use_behavioral_HDL=on  opt=Speed  use_embedded=on  optimum_pipeline=off  pipeline=on  use_rpm=on  placement_style=Rectangular shape  block_type=mult
      settings: xl_area=[0, 0, 0, 0, 0, 0, 0]  block_version=10.1.3
  Reinterpret4 : xbsIndex_r4/Reinterpret  force_arith_type=on  arith_type="Signed  (2's comp)"  force_bin_pt=on  bin_pt=7  block_type=reinterpret
      settings: infoedit="Changes signal type without altering the binary representation.   You can changed the signal between signed and unsigned, and relocate the binary point.<br><br>Hardware notes: In hardware this block costs nothing.<br><br>Example:  Suppose the input is 6 bits wide, signed, with 2 fractional bits, and the output is forced to unsigned with 0 fractional bits.  Then an input of -2.0 (1110.00 in binary 2's complement) becomes an output of 56 (111000 in binary)."  block_version=10.1.3
  Slice3 : xbsIndex_r4/Slice  nbits=8  boolean_output=off  mode=Lower Bit Location + Width  bit1=0  base1=MSB of Input  bit0=0  base0=LSB of Input  dbl_ovrd=off  block_type=slice
      settings: block_version=10.1.3
  Subsystem1 : Subsystem
  Subsystem2 : Subsystem
  Subsystem3 : Subsystem
  Subsystem4 : Subsystem
  Subsystem5 : Subsystem
  Subsystem6 : Subsystem
  Subsystem7 : Subsystem
  Subsystem8 : Subsystem
  bus_expand2 : Subsystem  AncestorBlock=casper_library_flow_control/bus_expand  mask(bus_expand){mode=divisions of equal size, outputNum=8, outputWidth=10, outputBinaryPt=0, outputArithmeticType=1, outputToWorkspace=off, variablePrefix=out, outputToModelAsWell=on}
      mask prompts: outputNum "Number of outputs:"; outputWidth "Output width:"; outputBinaryPt "Output binary point position:"; outputArithmeticType "Output arithmetic type: (Unsigned=0, Signed=1, Boolean=2)"; outputToWorkspace "Output to workspace?"; variablePrefix "Variable name prefix:"; outputToModelAsWell "Output to model as well?"
      mask help:
      | Expands a 'bus' made using a bus_create or Xilinx
      | concat block.
      | The input will be divided into the specified number
      | of outputs with the specified arithmetic types.
      | Divisions are made from most significant bit.
      mask init: same as test_r2_snapshot/10b_16b_cast/bus_expand2
      settings: AttributesFormatString=8 outputs
      mask StyleString: popup(divisions of equal size|divisions of arbitrary size),edit,edit,edit,edit,checkbox,edit,checkbox
      mask CallbackString: bus_expand_callback();||bus_expand_callback();|||bus_expand_callback();||
  trig : Outport
  wires:
  trig_pnt/1 -> Delay17/1
  bus_expand2/1(msb_out8) -> Subsystem1/1(din)
  bus_expand2/2(out7) -> Subsystem2/1(din)
  bus_expand2/3(out6) -> Subsystem3/1(din)
  bus_expand2/4(out5) -> Subsystem4/1(din)
  bus_expand2/5(out4) -> Subsystem5/1(din)
  bus_expand2/6(out3) -> Subsystem6/1(din)
  bus_expand2/7(out2) -> Subsystem7/1(din)
  bus_expand2/8(lsb_out1) -> Subsystem8/1(din)
  Subsystem1/1(trig) -> Logical1/1
  Subsystem2/1(trig) -> Logical1/2
  Subsystem3/1(trig) -> Logical1/3
  Subsystem4/1(trig) -> Logical1/4
  Subsystem5/1(trig) -> Logical1/5
  Subsystem6/1(trig) -> Logical1/6
  Subsystem7/1(trig) -> Logical1/7
  Subsystem8/1(trig) -> Logical1/8
  adc_data/1 -> bus_expand2/1(bus_in)
  Logical1/1 -> trig/1
  Mult/1 -> Subsystem7/2(thresh), Subsystem8/2(thresh), Subsystem6/2(thresh), Subsystem1/2(thresh), Subsystem2/2(thresh), Subsystem3/2(thresh), Subsystem4/2(thresh), Subsystem5/2(thresh)
  Reinterpret4/1 -> Mult/1, Mult/2
  Delay17/1 -> Slice3/1
  Slice3/1 -> Reinterpret4/1

== system test_r2_snapshot/trig1 ==
  adc_data : Inport
  trig_pnt : Inport  Port=2
  Delay17 : xbsIndex_r4/Delay  rst=off  infoeditControl=Selection of Reset will increase slice count due to use of real FFs and instead of SRLs  en=off  latency=2  dbl_ovrd=off  reg_retiming=on  block_type=delay
  Logical1 : xbsIndex_r4/Logical  logical_function=OR  inputs=8  en=off  latency=2  precision=Full  arith_type=Unsigned  n_bits=16  bin_pt=0  align_bp=on  dbl_ovrd=off  block_type=logical
  Mult : xbsIndex_r4/Mult  precision=Full  arith_type=Unsigned  n_bits=16  bin_pt=14  quantization=Truncate  overflow=Saturate  en=off  latency=4  dbl_ovrd=off  use_behavioral_HDL=on  opt=Speed  use_embedded=on  optimum_pipeline=off  pipeline=on  use_rpm=on  placement_style=Rectangular shape  block_type=mult
      settings: xl_area=[0, 0, 0, 0, 0, 0, 0]  block_version=10.1.3
  Reinterpret4 : xbsIndex_r4/Reinterpret  force_arith_type=on  arith_type="Signed  (2's comp)"  force_bin_pt=on  bin_pt=7  block_type=reinterpret
      settings: infoedit="Changes signal type without altering the binary representation.   You can changed the signal between signed and unsigned, and relocate the binary point.<br><br>Hardware notes: In hardware this block costs nothing.<br><br>Example:  Suppose the input is 6 bits wide, signed, with 2 fractional bits, and the output is forced to unsigned with 0 fractional bits.  Then an input of -2.0 (1110.00 in binary 2's complement) becomes an output of 56 (111000 in binary)."  block_version=10.1.3
  Slice3 : xbsIndex_r4/Slice  nbits=8  boolean_output=off  mode=Lower Bit Location + Width  bit1=0  base1=MSB of Input  bit0=0  base0=LSB of Input  dbl_ovrd=off  block_type=slice
      settings: block_version=10.1.3
  Subsystem1 : Subsystem
  Subsystem2 : Subsystem
  Subsystem3 : Subsystem
  Subsystem4 : Subsystem
  Subsystem5 : Subsystem
  Subsystem6 : Subsystem
  Subsystem7 : Subsystem
  Subsystem8 : Subsystem
  bus_expand2 : Subsystem  AncestorBlock=casper_library_flow_control/bus_expand  mask(bus_expand){mode=divisions of equal size, outputNum=8, outputWidth=10, outputBinaryPt=0, outputArithmeticType=1, outputToWorkspace=off, variablePrefix=out, outputToModelAsWell=on}
      mask prompts: outputNum "Number of outputs:"; outputWidth "Output width:"; outputBinaryPt "Output binary point position:"; outputArithmeticType "Output arithmetic type: (Unsigned=0, Signed=1, Boolean=2)"; outputToWorkspace "Output to workspace?"; variablePrefix "Variable name prefix:"; outputToModelAsWell "Output to model as well?"
      mask help:
      | Expands a 'bus' made using a bus_create or Xilinx
      | concat block.
      | The input will be divided into the specified number
      | of outputs with the specified arithmetic types.
      | Divisions are made from most significant bit.
      mask init: same as test_r2_snapshot/10b_16b_cast/bus_expand2
      settings: AttributesFormatString=8 outputs
      mask StyleString: popup(divisions of equal size|divisions of arbitrary size),edit,edit,edit,edit,checkbox,edit,checkbox
      mask CallbackString: bus_expand_callback();||bus_expand_callback();|||bus_expand_callback();||
  trig : Outport
  wires:
  Slice3/1 -> Reinterpret4/1
  Delay17/1 -> Slice3/1
  Reinterpret4/1 -> Mult/2, Mult/1
  Mult/1 -> Subsystem5/2(thresh), Subsystem4/2(thresh), Subsystem3/2(thresh), Subsystem2/2(thresh), Subsystem1/2(thresh), Subsystem6/2(thresh), Subsystem8/2(thresh), Subsystem7/2(thresh)
  Logical1/1 -> trig/1
  adc_data/1 -> bus_expand2/1(bus_in)
  Subsystem8/1(trig) -> Logical1/8
  Subsystem7/1(trig) -> Logical1/7
  Subsystem6/1(trig) -> Logical1/6
  Subsystem5/1(trig) -> Logical1/5
  Subsystem4/1(trig) -> Logical1/4
  Subsystem3/1(trig) -> Logical1/3
  Subsystem2/1(trig) -> Logical1/2
  Subsystem1/1(trig) -> Logical1/1
  bus_expand2/8(lsb_out1) -> Subsystem8/1(din)
  bus_expand2/7(out2) -> Subsystem7/1(din)
  bus_expand2/6(out3) -> Subsystem6/1(din)
  bus_expand2/5(out4) -> Subsystem5/1(din)
  bus_expand2/4(out5) -> Subsystem4/1(din)
  bus_expand2/3(out6) -> Subsystem3/1(din)
  bus_expand2/2(out7) -> Subsystem2/1(din)
  bus_expand2/1(msb_out8) -> Subsystem1/1(din)
  trig_pnt/1 -> Delay17/1

== system test_r2_snapshot/10b_16b_cast/adc0_bus_create1 ==
  in1 : Inport
  in2 : Inport  Port=2
  in3 : Inport  Port=3
  in4 : Inport  Port=4
  in5 : Inport  Port=5
  in6 : Inport  Port=6
  in7 : Inport  Port=7
  in8 : Inport  Port=8
  concatenate : xbsIndex_r4/Concat  num_inputs=8  dbl_ovrd=off  block_type=concat
  reinterpret{1..8} (8 alike) : xbsIndex_r4/Reinterpret  force_arith_type=on  arith_type=Unsigned  force_bin_pt=on  bin_pt=0  block_type=reinterpret
      settings: infoedit="Changes signal type without altering the binary representation.   You can changed the signal between signed and unsigned, and relocate the binary point.<br><br>Hardware notes: In hardware this block costs nothing.<br><br>Example:  Suppose the input is 6 bits wide, signed, with 2 fractional bits, and the output is forced to unsigned with 0 fractional bits.  Then an input of -2.0 (1110.00 in binary 2's complement) becomes an output of 56 (111000 in binary)."
  bus_out : Outport
  wires:
  reinterpret8/1 -> concatenate/8
  in8/1 -> reinterpret8/1
  reinterpret7/1 -> concatenate/7
  in7/1 -> reinterpret7/1
  reinterpret6/1 -> concatenate/6
  in6/1 -> reinterpret6/1
  reinterpret5/1 -> concatenate/5
  in5/1 -> reinterpret5/1
  reinterpret4/1 -> concatenate/4
  in4/1 -> reinterpret4/1
  reinterpret3/1 -> concatenate/3
  in3/1 -> reinterpret3/1
  reinterpret2/1 -> concatenate/2
  in2/1 -> reinterpret2/1
  reinterpret1/1 -> concatenate/1
  in1/1 -> reinterpret1/1
  concatenate/1 -> bus_out/1

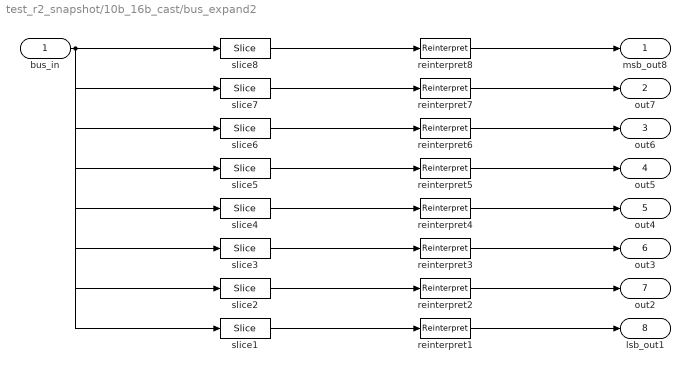
== system test_r2_snapshot/10b_16b_cast/bus_expand2 ==
  bus_in : Inport
  reinterpret{1..8} (8 alike) : xbsIndex_r4/Reinterpret  force_arith_type=on  arith_type="Signed  (2's comp)"  force_bin_pt=on  bin_pt=0  block_type=reinterpret
  slice1 : xbsIndex_r4/Slice  nbits=10  boolean_output=off  mode=Upper Bit Location + Width  bit1=-70  base1=MSB of Input  bit0=0  base0=LSB of Input  dbl_ovrd=off  block_type=slice
  slice2 : xbsIndex_r4/Slice  nbits=10  boolean_output=off  mode=Upper Bit Location + Width  bit1=-60  base1=MSB of Input  bit0=0  base0=LSB of Input  dbl_ovrd=off  block_type=slice
  slice3 : xbsIndex_r4/Slice  nbits=10  boolean_output=off  mode=Upper Bit Location + Width  bit1=-50  base1=MSB of Input  bit0=0  base0=LSB of Input  dbl_ovrd=off  block_type=slice
  slice4 : xbsIndex_r4/Slice  nbits=10  boolean_output=off  mode=Upper Bit Location + Width  bit1=-40  base1=MSB of Input  bit0=0  base0=LSB of Input  dbl_ovrd=off  block_type=slice
  slice5 : xbsIndex_r4/Slice  nbits=10  boolean_output=off  mode=Upper Bit Location + Width  bit1=-30  base1=MSB of Input  bit0=0  base0=LSB of Input  dbl_ovrd=off  block_type=slice
  slice6 : xbsIndex_r4/Slice  nbits=10  boolean_output=off  mode=Upper Bit Location + Width  bit1=-20  base1=MSB of Input  bit0=0  base0=LSB of Input  dbl_ovrd=off  block_type=slice
  slice7 : xbsIndex_r4/Slice  nbits=10  boolean_output=off  mode=Upper Bit Location + Width  bit1=-10  base1=MSB of Input  bit0=0  base0=LSB of Input  dbl_ovrd=off  block_type=slice
  slice8 : xbsIndex_r4/Slice  nbits=10  boolean_output=off  mode=Upper Bit Location + Width  bit1=0  base1=MSB of Input  bit0=0  base0=LSB of Input  dbl_ovrd=off  block_type=slice
  msb_out8 : Outport
  out7 : Outport  Port=2
  out6 : Outport  Port=3
  out5 : Outport  Port=4
  out4 : Outport  Port=5
  out3 : Outport  Port=6
  out2 : Outport  Port=7
  lsb_out1 : Outport  Port=8
  wires:
  bus_in/1 -> slice8/1, slice7/1, slice6/1, slice5/1, slice4/1, slice3/1, slice2/1, slice1/1
  slice8/1 -> reinterpret8/1
  reinterpret8/1 -> msb_out8/1
  slice7/1 -> reinterpret7/1
  reinterpret7/1 -> out7/1
  slice6/1 -> reinterpret6/1
  reinterpret6/1 -> out6/1
  slice5/1 -> reinterpret5/1
  reinterpret5/1 -> out5/1
  slice4/1 -> reinterpret4/1
  reinterpret4/1 -> out4/1
  slice3/1 -> reinterpret3/1
  reinterpret3/1 -> out3/1
  slice2/1 -> reinterpret2/1
  reinterpret2/1 -> out2/1
  slice1/1 -> reinterpret1/1
  reinterpret1/1 -> lsb_out1/1

== system test_r2_snapshot/10b_16b_cast1/adc0_bus_create1 ==
  in1 : Inport
  in2 : Inport  Port=2
  in3 : Inport  Port=3
  in4 : Inport  Port=4
  in5 : Inport  Port=5
  in6 : Inport  Port=6
  in7 : Inport  Port=7
  in8 : Inport  Port=8
  concatenate : xbsIndex_r4/Concat  num_inputs=8  dbl_ovrd=off  block_type=concat
  reinterpret{1..8} (8 alike) : xbsIndex_r4/Reinterpret  force_arith_type=on  arith_type=Unsigned  force_bin_pt=on  bin_pt=0  block_type=reinterpret
      settings: infoedit="Changes signal type without altering the binary representation.   You can changed the signal between signed and unsigned, and relocate the binary point.<br><br>Hardware notes: In hardware this block costs nothing.<br><br>Example:  Suppose the input is 6 bits wide, signed, with 2 fractional bits, and the output is forced to unsigned with 0 fractional bits.  Then an input of -2.0 (1110.00 in binary 2's complement) becomes an output of 56 (111000 in binary)."
  bus_out : Outport
  wires:
  concatenate/1 -> bus_out/1
  in1/1 -> reinterpret1/1
  reinterpret1/1 -> concatenate/1
  in2/1 -> reinterpret2/1
  reinterpret2/1 -> concatenate/2
  in3/1 -> reinterpret3/1
  reinterpret3/1 -> concatenate/3
  in4/1 -> reinterpret4/1
  reinterpret4/1 -> concatenate/4
  in5/1 -> reinterpret5/1
  reinterpret5/1 -> concatenate/5
  in6/1 -> reinterpret6/1
  reinterpret6/1 -> concatenate/6
  in7/1 -> reinterpret7/1
  reinterpret7/1 -> concatenate/7
  in8/1 -> reinterpret8/1
  reinterpret8/1 -> concatenate/8
